simulink model "heli_q8_lab2_controller"  (R2015b)
settings: Solver=ode1  StartTime=0.0  StopTime=inf  FixedStep=0.002  RelTol=1e-3
PostLoadFcn:
  | qc_set_target_type(getConfigSet(bdroot, 'QUARC Default Target Configuration'));
undefined symbols (not defined in the file): elev_lim, F, HIL, Joystick_gain_x, Joystick_gain_y, K, pitch_lim, qc_get_step_size, Vs0
libraries: quarc_library x4
settings Model: SimulationMode=external  ExtModeTrigDuration=30000  Creator=Rchan  LastModifiedBy=andregtu
settings SolverCC: PositivePriorityOrder=on
settings DataIOCC: SaveFormat=Array  SignalLoggingSaveFormat=ModelDataLogs
settings OptimizationCC: ExpressionDepthLimit=2147483647  InitFltsAndDblsToZero=on
settings DebuggingCC: SaveWithParameterizedLinksMsg=none  UnderspecifiedInitializationDetection=Classic  MergeDetectMultiDrivingBlocksExec=none  SolverPrmCheckMsg=warning  MultiTaskDSMMsg=warning  MultiTaskCondExecSysMsg=none  FcnCallInpInsideContextMsg=EnableAllAsWarning  StateNameClashWarn=warning
settings HardwareCC: ProdBitPerPointer=32  ProdLargestAtomicFloat=None  ProdIntDivRoundTo=Undefined  ProdEndianess=Unspecified  ProdWordSize=32  ProdHWDeviceType=32-bit Generic
settings RTWCC: SystemTargetFile=quarc_win64.tlc  TemplateMakefile=quarc_default_tmf  Description=QUARC Win64 Target
settings GRTTargetCC: ParMdlRefBuildCompliant=off  CompOptLevelCompliant=off  GeneratePreprocessorConditionals=Disable all  CombineOutputUpdateFcns=off  MatFileLogging=off  GRTInterface=on  UseToolchainInfoCompliant=off  ExtMode=on  ExtModeMexFile=quarc_comm
settings ConfigComp: CovModelRefEnable=Off  CovSFcnEnable=off

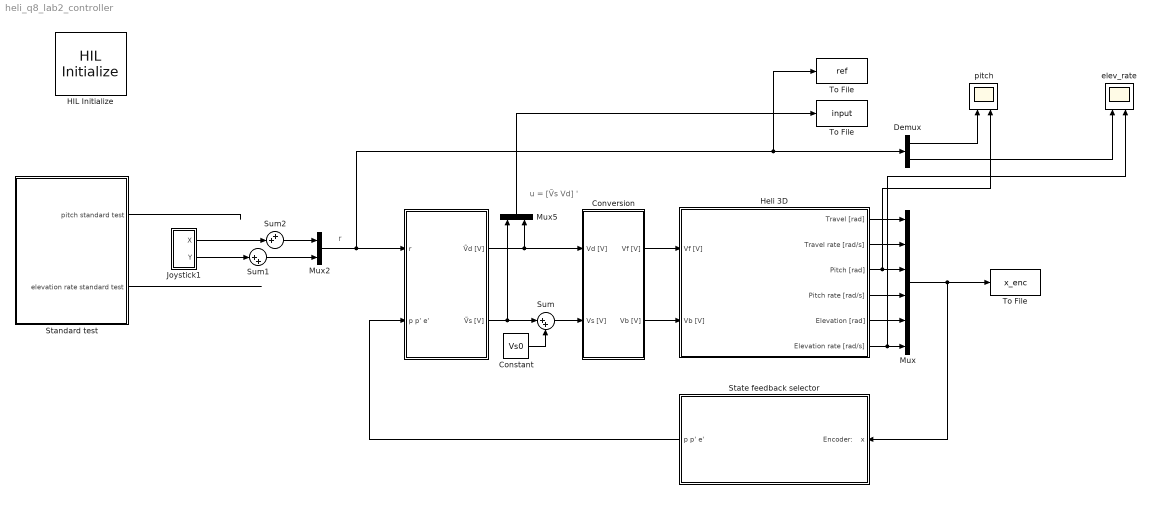
== system heli_q8_lab2_controller ==
  note: r
  note: u = [Ṽs Vd] '
  "  " : Subsystem
  Constant : Constant  Value=Vs0
  Conversion : Subsystem
  Demux : Demux  Outputs=2
  HIL Initialize : quarc_library/Data Acquisition/Generic/Configuration/HIL Initialize  Priority=-99  object_name=HIL-1  board_type=q8_usb  board_number=0  board_options=update_rate=normal;decimation=1  exclusive=off  active=off  hardware_clocks=[0:2]  clock_modes=[]  initial_clock_frequencies=[]  set_clock_params_at_start=off  set_clock_params_at_switch_in=off  set_clock_frequencies_at_start=off  set_clock_frequencies_at_switch_in=off  analog_input_channels=[0:7]  analog_input_maximums=10  analog_input_minimums=-10  set_analog_input_params_at_start=on  set_analog_input_params_at_switch_in=off  analog_output_channels=[0:7]  analog_output_maximums=10  analog_output_minimums=-10  initial_analog_outputs=[0]  final_analog_outputs=[0]  watchdog_analog_outputs=0  set_analog_output_params_at_start=on  set_analog_output_params_at_switch_in=off  set_analog_outputs_at_start=on  set_analog_outputs_at_switch_in=off  set_analog_outputs_at_terminate=on  set_analog_outputs_at_switch_out=off  set_analog_outputs_on_watchdog=off  digital_input_channels=[]  digital_output_channels=[]  digital_output_configuration=[]  initial_digital_outputs=[1]  final_digital_outputs=[1]  watchdog_digital_outputs=[1]  set_digital_output_params_at_start=off  set_digital_output_params_at_switch_in=off  set_digital_outputs_at_start=on  set_digital_outputs_at_switch_in=off  set_digital_outputs_at_terminate=on  set_digital_outputs_at_switch_out=off  set_digital_outputs_on_watchdog=off  encoder_channels=[0:7]  quadrature=[4]  encoder_filter_frequency=[]  initial_encoder_counts=[0]  set_encoder_params_at_start=on  set_encoder_params_at_switch_in=off  set_encoder_counts_at_start=on  set_encoder_counts_at_switch_in=off  pwm_channels=[0:7]  pwm_modes=0  pwm_frequency=99.532799999999995e6/4095  pwm_configuration=[0]  pwm_alignment=[0]  pwm_polarity=[1]  pwm_leading_deadband=[0]  pwm_trailing_deadband=[0]  initial_pwm_outputs=[0]  final_pwm_outputs=[0]  watchdog_pwm_outputs=[0]  set_pwm_params_at_start=on  set_pwm_params_at_switch_in=off  set_pwm_outputs_at_start=on  set_pwm_outputs_at_switch_in=off  set_pwm_outputs_at_terminate=on  set_pwm_outputs_at_switch_out=off  set_pwm_outputs_on_watchdog=off  other_output_channels=[]  initial_other_outputs=[]  final_other_outputs=[]  watchdog_other_outputs=[]  set_other_outputs_at_start=off  set_other_outputs_at_switch_in=off  set_other_outputs_at_terminate=off  set_other_outputs_at_switch_out=off  set_other_outputs_on_watchdog=off
  Heli 3D : Subsystem
  Joystick1 : Subsystem
  Mux : Mux  Inputs=6
  Mux2 : Mux  Inputs=2
  Mux5 : Mux  Inputs=2
  Standard test : Subsystem
  State feedback selector : Subsystem
  Sum : Sum  Inputs=|++
  Sum1 : Sum  Inputs=|++
  Sum2 : Sum  Inputs=++|
  To File : ToFile  Filename=x_enc
  "To File   " : ToFile  Filename=ref
  "To File    " : ToFile  Filename=input
  "elev_rate " : Scope  NumInputPorts=2
  pitch : Scope  NumInputPorts=2
  wires:
  Conversion/2(Vb [V]) -> Heli 3D/2(Vb [V])
  Conversion/1(Vf [V]) -> Heli 3D/1(Vf [V])
  Heli 3D/1(Travel [rad]) -> Mux/1
  Heli 3D/2(Travel rate [rad/s]) -> Mux/2
  Heli 3D/4(Pitch rate [rad/s]) -> Mux/4
  Heli 3D/5(Elevation [rad]) -> Mux/5
  Mux/1 -> State feedback selector/1(Encoder:    x), To File/1
  Constant/1 -> Sum/2
  Sum/1 -> Conversion/2(Vs [V])
  State feedback selector/1(p p' e') -> "  "/2(p p' e')
  Joystick1/1(X) -> Sum2/2
  Joystick1/2(Y) -> Sum1/1
  Sum1/1 -> Mux2/2
  Sum2/1 -> Mux2/1
  Standard test/1(pitch standard test) -> ?
  Standard test/2(elevation rate standard test) -> ?
  Heli 3D/3(Pitch [rad]) -> Mux/3, pitch/2
  Mux2/1 -> "To File   "/1, Demux/1, "  "/1(r)
  Demux/1 -> pitch/1
  "  "/2(Ṽs [V]) -> Mux5/1, Sum/1
  "  "/1(Ṽd [V]) -> Conversion/1(Vd [V]), Mux5/2
  Mux5/1 -> "To File    "/1
  Heli 3D/6(Elevation rate [rad/s]) -> "elev_rate "/2, Mux/6
  Demux/2 -> "elev_rate "/1

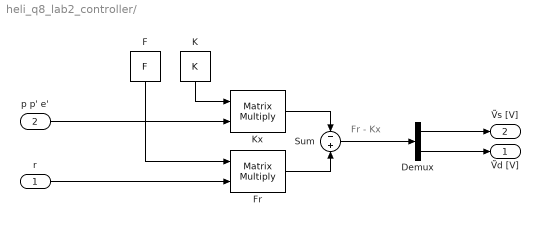
== system heli_q8_lab2_controller/   ==
  note: Fr - Kx
  r : Inport
  p p' e' : Inport  Port=2
  Demux : Demux  Outputs=2
  F : Constant  Value=F  VectorParams1D=off
  Fr : Product  Multiplication=Matrix(*)
  K : Constant  Value=K  VectorParams1D=off
  Kx : Product  Multiplication=Matrix(*)  RndMeth=Nearest  OutDataTypeStr=Inherit: Same as first input
  Sum : Sum  Inputs=-|+
  Ṽd [V] : Outport  InitialOutput=0
  Ṽs [V] : Outport  Port=2  InitialOutput=0
  wires:
  K/1 -> Kx/1
  F/1 -> Fr/1
  Fr/1 -> Sum/2
  Kx/1 -> Sum/1
  Sum/1 -> Demux/1
  Demux/1 -> Ṽs [V]/1
  Demux/2 -> Ṽd [V]/1
  r/1 -> Fr/2
  p p' e'/1 -> Kx/2

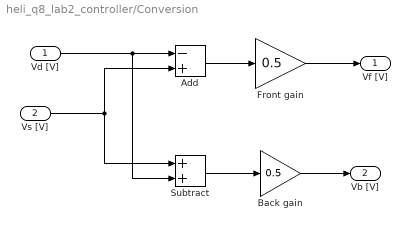
== system heli_q8_lab2_controller/Conversion ==
  Vd [V] : Inport
  Vs [V] : Inport  Port=2
  Add : Sum  Inputs=-+
  Back gain : Gain  Gain=0.5
  Front gain : Gain  Gain=0.5
  Subtract : Sum
  Vf [V] : Outport
  Vb [V] : Outport  Port=2
  wires:
  Vd [V]/1 -> Subtract/2, Add/1
  Vs [V]/1 -> Subtract/1, Add/2
  Subtract/1 -> Back gain/1
  Back gain/1 -> Vb [V]/1
  Add/1 -> Front gain/1
  Front gain/1 -> Vf [V]/1

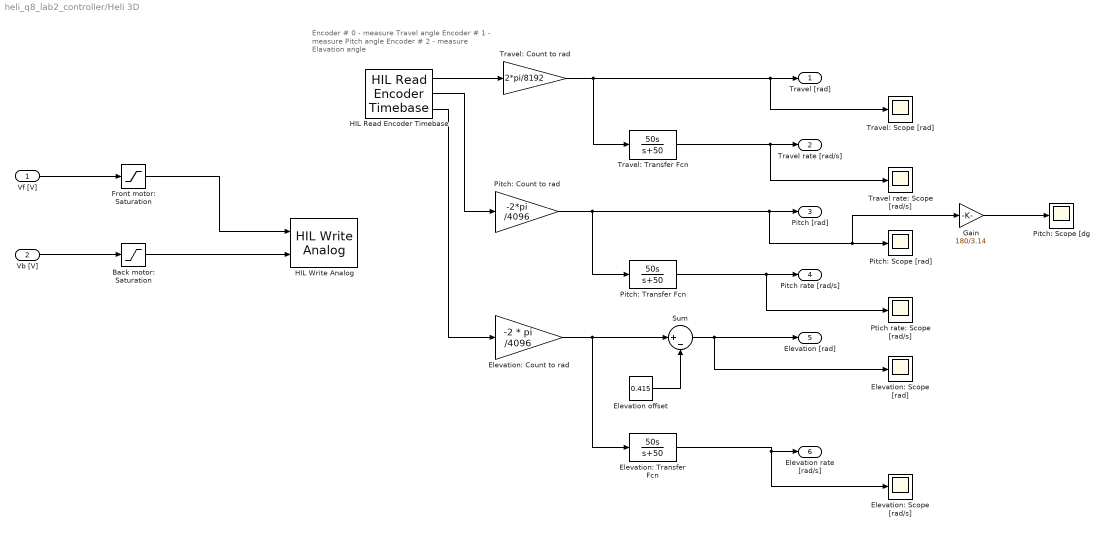
== system heli_q8_lab2_controller/Heli 3D ==
  note: Encoder # 0 - measure Travel angle
      | Encoder # 1 - measure Pitch angle
      | Encoder # 2 - measure Elavation angle
  Vf [V] : Inport
  Vb [V] : Inport  Port=2
  Back motor: Saturation : Saturate  UpperLimit=5  LowerLimit=-5
  Elevation offset : Constant  Value=0.415
  Elevation: Count to rad : Gain  Gain=-2 * pi /4096
  Elevation: Scope [rad/s] : Scope
  Elevation: Scope [rad] : Scope
  Elevation: Transfer Fcn : TransferFcn  Numerator=[50 0]  Denominator=[1 50]
  Front motor: Saturation : Saturate  UpperLimit=5  LowerLimit=-5
  Gain : Gain  Gain=180/3.14
  HIL Read Encoder Timebase : quarc_library/Data Acquisition/Generic/Timebases/HIL Read Encoder Timebase  object_name=HIL-1  clock=0  channels=[0:2]  samples_in_buffer=max(ceil(1/qc_get_step_size), 1)  active=on  vector_output=off  data_type_mode=Inherit via back propagation  data_type=double
  HIL Write Analog : quarc_library/Data Acquisition/Generic/Immediate I//O/HIL Write Analog  object_name=HIL-1  channels=[0:1]  sample_time=-1  active=off  vector_input=off
  Pitch: Count to rad : Gain  Gain=-2*pi /4096
  Pitch: Scope [dg : Scope
  Pitch: Scope [rad] : Scope
  Pitch: Transfer Fcn : TransferFcn  Numerator=[50 0]  Denominator=[1 50]
  Ptich rate: Scope [rad/s] : Scope
  Sum : Sum  Inputs=|+-
  Travel rate: Scope [rad/s] : Scope
  Travel: Count to rad : Gain  Gain=2*pi/8192
  Travel: Scope [rad] : Scope
  Travel: Transfer Fcn : TransferFcn  Numerator=[50 0]  Denominator=[1 50]
  Travel [rad] : Outport
  Travel rate [rad/s] : Outport  Port=2
  Pitch [rad] : Outport  Port=3
  Pitch rate [rad/s] : Outport  Port=4
  Elevation [rad] : Outport  Port=5
  Elevation rate [rad/s] : Outport  Port=6
  wires:
  HIL Read Encoder Timebase/1 -> Travel: Count to rad/1
  HIL Read Encoder Timebase/2 -> Pitch: Count to rad/1
  HIL Read Encoder Timebase/3 -> Elevation: Count to rad/1
  Travel: Count to rad/1 -> Travel: Scope [rad]/1, Travel [rad]/1, Travel: Transfer Fcn/1
  Travel: Transfer Fcn/1 -> Travel rate: Scope [rad/s]/1, Travel rate [rad/s]/1
  Pitch: Count to rad/1 -> Pitch: Transfer Fcn/1, Gain/1, Pitch: Scope [rad]/1, Pitch [rad]/1
  Pitch: Transfer Fcn/1 -> Ptich rate: Scope [rad/s]/1, Pitch rate [rad/s]/1
  Elevation: Count to rad/1 -> Sum/1, Elevation: Transfer Fcn/1
  Elevation: Transfer Fcn/1 -> Elevation: Scope [rad/s]/1, Elevation rate [rad/s]/1
  Vf [V]/1 -> Front motor: Saturation/1
  Vb [V]/1 -> Back motor: Saturation/1
  Front motor: Saturation/1 -> HIL Write Analog/1
  Back motor: Saturation/1 -> HIL Write Analog/2
  Elevation offset/1 -> Sum/2
  Sum/1 -> Elevation: Scope [rad]/1, Elevation [rad]/1
  Gain/1 -> Pitch: Scope [dg/1

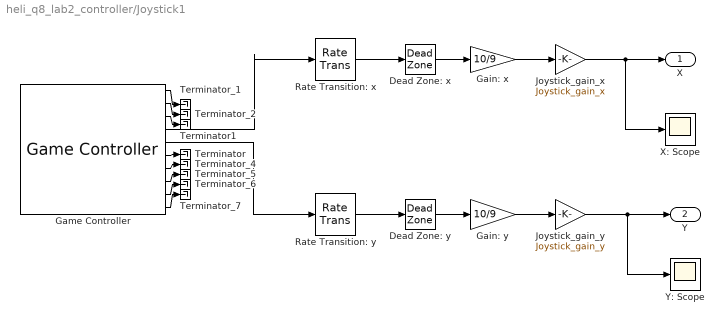
== system heli_q8_lab2_controller/Joystick1 ==
  Dead Zone: x : DeadZone  LowerValue=-0.1  UpperValue=0.1  SaturateOnIntegerOverflow=on
  Dead Zone: y : DeadZone  LowerValue=-0.1  UpperValue=0.1  SaturateOnIntegerOverflow=on
  Gain: x : Gain  Gain=10/9
  Gain: y : Gain  Gain=10/9
  Game Controller : quarc_library/Devices/Peripherals/Target/Game Controller  controller=1  buffer_size=12  deadzone=[]  saturation=[]  sample_time=max(qc_get_step_size, 0.01)  auto_center=off  enabled=on
  Joystick_gain_x : Gain  Gain=Joystick_gain_x
  Joystick_gain_y : Gain  Gain=Joystick_gain_y
  Rate Transition: x : RateTransition
  Rate Transition: y : RateTransition
  Terminator : Terminator
  Terminator1 : Terminator
  Terminator_{1..2,4..7} (6 alike) : Terminator
  X: Scope : Scope
  Y: Scope : Scope
  X : Outport
  Y : Outport  Port=2
  wires:
  Joystick_gain_y/1 -> Y/1, Y: Scope/1
  Joystick_gain_x/1 -> X: Scope/1, X/1
  Gain: y/1 -> Joystick_gain_y/1
  Gain: x/1 -> Joystick_gain_x/1
  Dead Zone: y/1 -> Gain: y/1
  Dead Zone: x/1 -> Gain: x/1
  Game Controller/6 -> Terminator/1
  Game Controller/3 -> Terminator1/1
  Game Controller/10 -> Terminator_7/1
  Game Controller/9 -> Terminator_6/1
  Game Controller/8 -> Terminator_5/1
  Game Controller/7 -> Terminator_4/1
  Game Controller/2 -> Terminator_2/1
  Game Controller/1 -> Terminator_1/1
  Game Controller/4 -> Rate Transition: x/1
  Game Controller/5 -> Rate Transition: y/1
  Rate Transition: x/1 -> Dead Zone: x/1
  Rate Transition: y/1 -> Dead Zone: y/1

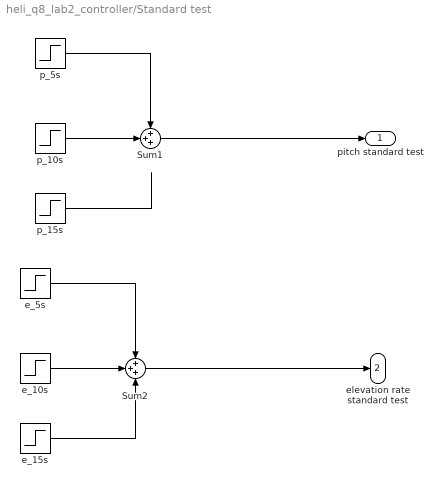
== system heli_q8_lab2_controller/Standard test ==
  Sum1 : Sum  Inputs=3
  Sum2 : Sum  Inputs=3
  e_10s : Step  Time=8  After=elev_lim  SampleTime=0
  e_15s : Step  Time=12  After=-elev_lim/2  SampleTime=0
  e_5s : Step  Time=4  Before=elev_lim  After=-elev_lim/2  SampleTime=0
  p_10s : Step  Time=8  After=-pitch_lim  SampleTime=0
  p_15s : Step  Time=12  After=-pitch_lim  SampleTime=0
  p_5s : Step  Time=4  After=pitch_lim  SampleTime=0
  pitch standard test : Outport
  elevation rate standard test : Outport  Port=2
  wires:
  Sum1/1 -> pitch standard test/1
  p_10s/1 -> Sum1/2
  p_5s/1 -> Sum1/1
  p_15s/1 -> ?
  Sum2/1 -> elevation rate standard test/1
  e_5s/1 -> Sum2/1
  e_10s/1 -> Sum2/2
  e_15s/1 -> Sum2/3

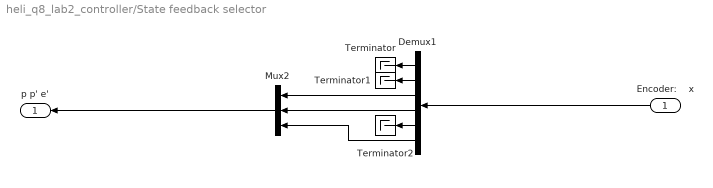
== system heli_q8_lab2_controller/State feedback selector ==
  Encoder:    x : Inport
  Demux1 : Demux  Outputs=6
  Mux2 : Mux  Inputs=3
  Terminator : Terminator
  Terminator1 : Terminator
  Terminator2 : Terminator
  p p' e' : Outport
  wires:
  Encoder:    x/1 -> Demux1/1
  Demux1/3 -> Mux2/1
  Demux1/4 -> Mux2/2
  Demux1/6 -> Mux2/3
  Mux2/1 -> p p' e'/1
  Demux1/1 -> Terminator/1
  Demux1/2 -> Terminator1/1
  Demux1/5 -> Terminator2/1
